simulink model "lab3_robotika_model"  (R2016a)
settings: Solver=VariableStepAuto  StartTime=0.0  StopTime=10  FixedStep=0.001  RelTol=1e-3
undefined symbols (not defined in the file): init, input
libraries: roblocks x12
settings Model: Creator=pc  LastModifiedBy=pc

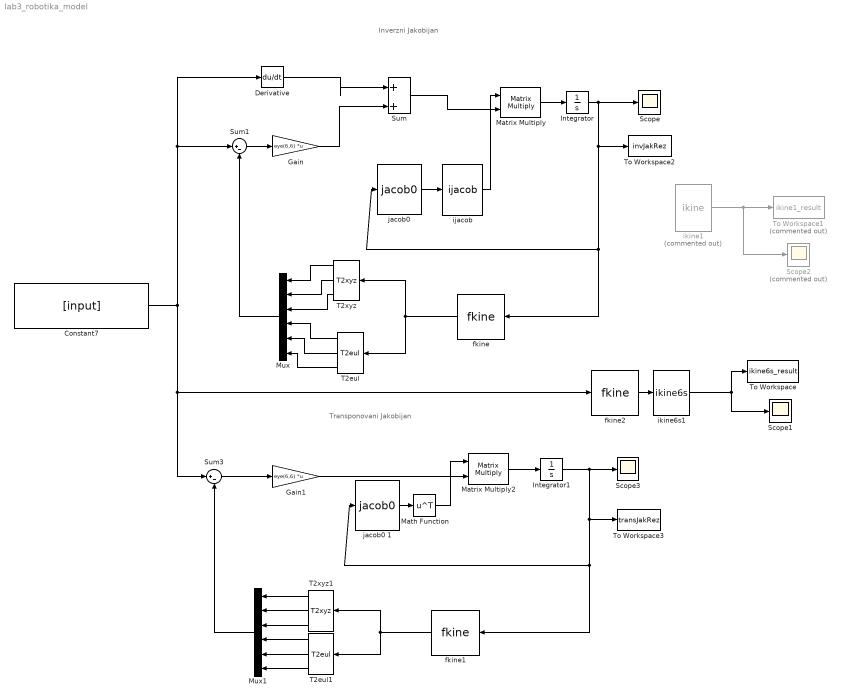
== system lab3_robotika_model ==
  note: Transponovani Jakobijan
  note: Inverzni Jakobijan
  Constant7 : Constant  Value=[input]
  Derivative : Derivative
  Gain : Gain  Gain=eye(6,6)  Multiplication=Matrix(K*u)
  Gain1 : Gain  Gain=eye(6,6)  Multiplication=Matrix(K*u)
  Integrator : Integrator  InitialCondition=init
  Integrator1 : Integrator
  Math Function : Math  Operator=transpose  SaturateOnIntegerOverflow=on
  Matrix Multiply : Product  Multiplication=Matrix(*)
  Matrix Multiply2 : Product  Multiplication=Matrix(*)
  Mux : Mux  Inputs=6
  Mux1 : Mux  Inputs=6
  Scope : Scope
  Scope1 : Scope
  Scope2 : Scope  Commented=on
  Scope3 : Scope
  Sum : Sum  Inputs=|++
  Sum1 : Sum  Inputs=|+-
  Sum3 : Sum  Inputs=|+-
  T2eul : roblocks/Transform Conversion/T2eul
  T2eul1 : roblocks/Transform Conversion/T2eul
  T2xyz : roblocks/Transform Conversion/T2xyz
  T2xyz1 : roblocks/Transform Conversion/T2xyz
  To Workspace : ToWorkspace  VariableName=ikine6s_result  SampleTime=-1
  To Workspace1 : ToWorkspace  Commented=on  VariableName=ikine1_result  SaveFormat=Timeseries  SampleTime=-1
  To Workspace2 : ToWorkspace  VariableName=invJakRez  SampleTime=-1
  To Workspace3 : ToWorkspace  VariableName=transJakRez  SampleTime=-1
  fkine : roblocks/Kinematics/fkine  robot=p560
  fkine1 : roblocks/Kinematics/fkine  robot=p560
  fkine2 : roblocks/Kinematics/fkine  robot=p560
  ijacob : roblocks/Kinematics/ijacob
  ikine1 : roblocks/Kinematics/ikine  Commented=on  robot=p560  q0=[0 0 0 0 0 0]  M=[1 1 1 1 1 1]  pinv=off  options={}
  ikine6s1 : roblocks/Kinematics/ikine6s  robot=p560  conf='rdf'
  "jacob0 " : roblocks/Kinematics/jacob0   robot=p560
  jacob0 1 : roblocks/Kinematics/jacob0   robot=p560
  wires:
  ikine1/1 -> Scope2/1, To Workspace1/1
  ikine6s1/1 -> Scope1/1, To Workspace/1
  "jacob0 "/1 -> ijacob/1
  Integrator/1 -> "jacob0 "/1, fkine/1, To Workspace2/1, Scope/1
  Matrix Multiply/1 -> Integrator/1
  Derivative/1 -> Sum/1
  Sum1/1 -> Gain/1
  Gain/1 -> Sum/2
  fkine/1 -> T2eul/1, T2xyz/1
  Mux/1 -> Sum1/2
  T2xyz/1 -> Mux/1
  T2xyz/2 -> Mux/2
  T2xyz/3 -> Mux/3
  T2eul/1 -> Mux/4
  T2eul/2 -> Mux/5
  T2eul/3 -> Mux/6
  Constant7/1 -> fkine2/1, Sum3/1, Derivative/1, Sum1/1
  jacob0 1/1 -> Math Function/1
  Integrator1/1 -> Scope3/1, jacob0 1/1, fkine1/1, To Workspace3/1
  Matrix Multiply2/1 -> Integrator1/1
  Math Function/1 -> Matrix Multiply2/1
  Sum3/1 -> Gain1/1
  fkine1/1 -> T2eul1/1, T2xyz1/1
  Mux1/1 -> Sum3/2
  T2xyz1/1 -> Mux1/1
  T2xyz1/2 -> Mux1/2
  T2xyz1/3 -> Mux1/3
  T2eul1/1 -> Mux1/4
  T2eul1/2 -> Mux1/5
  T2eul1/3 -> Mux1/6
  Gain1/1 -> Matrix Multiply2/2
  ijacob/1 -> Matrix Multiply/1
  Sum/1 -> Matrix Multiply/2
  fkine2/1 -> ikine6s1/1
